simulink model "ZT_VehCtrl_18B"  (R2018b)
settings: Solver=FixedStepAuto  StartTime=0.0  StopTime=inf  FixedStep=0.005  RelTol=1e-3
InitFcn:
  | mbd_mpc_consistency_checks(bdroot(gcs));
undefined symbols (not defined in the file or in its folder): ANG_DEAD, BMS_NormalPwr, BrkPrsByBrkPct_TB_X, BrkPrsByBrkPct_TB_Y, DELAY_DISCHARGE, DELAY_RCUOFF, DRV_BACKWARD, DRV_BRAKE, DRV_FORWARD, DRV_NEUTRAL, DRV_PARK, DRV_UNPARK, DRV_ZEROTURN, EPB_LOCK, EPB_UNLOCK, ExtraLoadPwr, FanOff, fifo_0_vect, fifo_1_vect, HiFanReq, HV_finished, HV_No_Active, HV_POWER_OFF, HV_POWER_ON, HVDown, HVON, KaTLS_v_DrgUp_X_VehSpd, KeFTM_s_Way1OffDlyTime, KeFTM_TK_Way1CoolLv2OffBatTemp, KeFTM_TK_Way1CoolLv2OffMtrTemp, KeFTM_TK_Way1CoolLv2OnBatTemp, KeFTM_TK_Way1CoolLv2OnMtrTemp, KeFTM_TK_Way1CoolLv3OffBatTemp, KeFTM_TK_Way1CoolLv3OffMtrTemp, KeFTM_TK_Way1CoolLv3OnBatTemp, KeFTM_TK_Way1CoolLv3OnMtrTemp, KeFTM_TK_Way1CoolLv4OffBatTemp, KeFTM_TK_Way1CoolLv4OffMtrTemp, KeFTM_TK_Way1CoolLv4OnBatTemp, KeFTM_TK_Way1CoolLv4OnMtrTemp, Kp1, Kp2, LowFanReq, LQFP, MtrPwrFactor_RCU, MtrPwrHighToMidThd, MtrPwrLowToMidThd, MtrPwrMidToHighThd, MtrPwrMidToLowThd, MtrTrqMax, PCT_DEAD, Precharge, PTO_1000, PTO_540, pts1_fifo_0_vect, pts1_fifo_1_vect, pts2_fifo_0_vect, pts2_fifo_1_vect, pts3_fifo_0_vect, pts3_fifo_1_vect ... (+24)
libraries: mbd_mpc574x_ec_toolbox x173, canmsglib x72, simulink x57
(part 5 of 12)

== system ZT_VehCtrl_18B/Initialization & SPI timer1/CS5 LS/Subsystem ==
  Data Store Read : DataStoreRead  DataStoreName=SPIO_CS1_InitFlg
  Merge : Merge  Inputs=3
  Merge1 : Merge  Inputs=3
  SPI_en : Subsystem  TreatAsAtomicUnit=on
  Switch Case : SwitchCase  CaseConditions={1,2,3}  ShowDefaultCase=off
  "clear " : Subsystem  TreatAsAtomicUnit=on
  confi_enbit : Subsystem  TreatAsAtomicUnit=on
  Out1 : Outport
  Out2 : Outport  Port=2
  wires:
  confi_enbit/1(Out1) -> Merge/3
  SPI_en/1(Out1) -> Merge/2
  "clear "/2(Out2) -> Merge1/1
  confi_enbit/2(Out2) -> Merge1/3
  "clear "/1(Out1) -> Merge/1
  Switch Case/1 -> "clear "/Action
  Switch Case/3 -> confi_enbit/Action
  Merge1/1 -> Out2/1
  Switch Case/2 -> SPI_en/Action
  SPI_en/2(Out2) -> Merge1/2
  Data Store Read/1 -> Switch Case/1
  Merge/1 -> Out1/1

== system ZT_VehCtrl_18B/SPI_EEPROM/SPI_write/SPI_enable ==
  Action Port : ActionPort
  Constant1 : Constant  Value=2
  Data Store Write : DataStoreWrite  DataStoreName=Write_Ctrl
  Data Type Conversion : DataTypeConversion  OutDataTypeStr=uint8
  Data Type Conversion3 : DataTypeConversion
  Data Type Conversion8 : DataTypeConversion
  Demux1 : Demux  Outputs=1
  SPI_Master_Transfer_To1 : mbd_mpc574x_ec_toolbox/Communication Blocks/SPI Blocks/SPI_Master_Transfer  Priority=2  InstanceNumber=0  xfermode=Non blocking  timeout=50  spi_upd=on  WhichPCS=0
  Terminator : Terminator
  Vector Concatenate1 : Concatenate  NumInputs=1
  write_enable : Constant  Value=6  OutDataTypeStr=uint8
  wires:
  Data Type Conversion3/1 -> Terminator/1  "r8"
  SPI_Master_Transfer_To1/1 -> Demux1/1
  Demux1/1 -> Data Type Conversion3/1
  Vector Concatenate1/1 -> SPI_Master_Transfer_To1/1
  write_enable/1 -> Data Type Conversion/1
  Data Type Conversion/1 -> Vector Concatenate1/1  "d8"
  Constant1/1 -> Data Type Conversion8/1
  Data Type Conversion8/1 -> Data Store Write/1

== system ZT_VehCtrl_18B/SPI_EEPROM/SPI_write/SPI_write ==
  Action Port : ActionPort
  "Address_High " : Constant  Value=hex2dec('FF')  OutDataTypeStr=uint8
  Address_Low : Constant  Value=hex2dec('FF')
  Constant1 : Constant
  Data Store Read : DataStoreRead  DataStoreName=A_write
  Data Store Write : DataStoreWrite  DataStoreName=Write_Ctrl
  Data Type Conversion{,1..2,5} (4 alike) : DataTypeConversion  OutDataTypeStr=uint8
  Data Type Conversion{3..4,6..8} (5 alike) : DataTypeConversion
  Demux1 : Demux
  SPI_Master_Transfer_To1 : mbd_mpc574x_ec_toolbox/Communication Blocks/SPI Blocks/SPI_Master_Transfer  Priority=2  InstanceNumber=0  xfermode=Non blocking  timeout=50  spi_upd=on  WhichPCS=0
  Terminator{,1..3} (4 alike) : Terminator
  Vector Concatenate1 : Concatenate  NumInputs=4
  write_set : Constant  Value=2  OutDataTypeStr=uint8
  wires:
  Data Type Conversion4/1 -> Terminator1/1  "r5"
  Data Type Conversion3/1 -> Terminator/1  "r4"
  SPI_Master_Transfer_To1/1 -> Demux1/1
  Demux1/1 -> Data Type Conversion3/1
  Vector Concatenate1/1 -> SPI_Master_Transfer_To1/1
  Demux1/2 -> Data Type Conversion4/1
  Address_Low/1 -> Data Type Conversion5/1
  Data Type Conversion/1 -> Vector Concatenate1/1  "d4"
  Data Type Conversion1/1 -> Vector Concatenate1/2  "d5"
  write_set/1 -> Data Type Conversion/1
  "Address_High "/1 -> Data Type Conversion1/1
  Data Store Read/1 -> Data Type Conversion2/1
  Constant1/1 -> Data Type Conversion8/1
  Data Type Conversion5/1 -> Vector Concatenate1/3  "d6"
  Data Type Conversion2/1 -> Vector Concatenate1/4  "d7"
  Data Type Conversion6/1 -> Terminator2/1  "r6"
  Demux1/3 -> Data Type Conversion6/1
  Data Type Conversion7/1 -> Terminator3/1  "r7"
  Demux1/4 -> Data Type Conversion7/1
  Data Type Conversion8/1 -> Data Store Write/1

== system ZT_VehCtrl_18B/SigIn/CAN0 /BMS Cell Battery Temperature ==
  ID : Inport
  Data : Inport  Port=2
  length : Inport  Port=3
  timestamp : Inport  Port=4
  Switch Case : SwitchCase  CaseConditions={hex2dec('357')}  ShowDefaultCase=off
  UNPACK : Subsystem  TreatAsAtomicUnit=on
  Message : Outport
  wires:
  UNPACK/1(Message) -> Message/1
  length/1 -> UNPACK/3(length)
  timestamp/1 -> UNPACK/4(timestamp)
  Data/1 -> UNPACK/2(data)
  ID/1 -> Switch Case/1, UNPACK/1(ID)
  Switch Case/1 -> UNPACK/Action

== system ZT_VehCtrl_18B/SigIn/CAN0 /BMS Cell HeatingTemperature ==
  ID : Inport
  Data : Inport  Port=2
  length : Inport  Port=3
  timestamp : Inport  Port=4
  Switch Case : SwitchCase  CaseConditions={hex2dec('3F3')}  ShowDefaultCase=off
  UNPACK : Subsystem  TreatAsAtomicUnit=on
  Message : Outport
  wires:
  Switch Case/1 -> UNPACK/Action
  ID/1 -> UNPACK/1(ID), Switch Case/1
  Data/1 -> UNPACK/2(data)
  timestamp/1 -> UNPACK/4(timestamp)
  length/1 -> UNPACK/3(length)
  UNPACK/1(Message) -> Message/1

== system ZT_VehCtrl_18B/SigIn/CAN0 /BMS Cell Pole Temperature ==
  ID : Inport
  Data : Inport  Port=2
  length : Inport  Port=3
  timestamp : Inport  Port=4
  Switch Case : SwitchCase  CaseConditions={hex2dec('3F4')}  ShowDefaultCase=off
  UNPACK : Subsystem  TreatAsAtomicUnit=on
  Message : Outport
  wires:
  UNPACK/1(Message) -> Message/1
  length/1 -> UNPACK/3(length)
  timestamp/1 -> UNPACK/4(timestamp)
  Data/1 -> UNPACK/2(data)
  ID/1 -> Switch Case/1, UNPACK/1(ID)
  Switch Case/1 -> UNPACK/Action

== system ZT_VehCtrl_18B/SigIn/CAN0 /BMS Cell Voltage Infor ==
  ID : Inport
  Data : Inport  Port=2
  length : Inport  Port=3
  timestamp : Inport  Port=4
  Switch Case : SwitchCase  CaseConditions={hex2dec('356')}  ShowDefaultCase=off
  UNPACK : Subsystem  TreatAsAtomicUnit=on
  Message : Outport
  wires:
  UNPACK/1(Message) -> Message/1
  length/1 -> UNPACK/3(length)
  timestamp/1 -> UNPACK/4(timestamp)
  Data/1 -> UNPACK/2(data)
  ID/1 -> Switch Case/1, UNPACK/1(ID)
  Switch Case/1 -> UNPACK/Action

== system ZT_VehCtrl_18B/SigIn/CAN0 /BMS CumuCap Infor ==
  ID : Inport
  Data : Inport  Port=2
  length : Inport  Port=3
  timestamp : Inport  Port=4
  Switch Case : SwitchCase  CaseConditions={hex2dec('3F5')}  ShowDefaultCase=off
  UNPACK : Subsystem  TreatAsAtomicUnit=on
  Message : Outport
  wires:
  Switch Case/1 -> UNPACK/Action
  ID/1 -> UNPACK/1(ID), Switch Case/1
  Data/1 -> UNPACK/2(data)
  timestamp/1 -> UNPACK/4(timestamp)
  length/1 -> UNPACK/3(length)
  UNPACK/1(Message) -> Message/1

== system ZT_VehCtrl_18B/SigIn/CAN0 /BMS CumuTimeInfor1 ==
  ID : Inport
  Data : Inport  Port=2
  length : Inport  Port=3
  timestamp : Inport  Port=4
  Switch Case : SwitchCase  CaseConditions={hex2dec('203')}  ShowDefaultCase=off
  UNPACK : Subsystem  TreatAsAtomicUnit=on
  Message : Outport
  wires:
  UNPACK/1(Message) -> Message/1
  length/1 -> UNPACK/3(length)
  timestamp/1 -> UNPACK/4(timestamp)
  Data/1 -> UNPACK/2(data)
  ID/1 -> Switch Case/1, UNPACK/1(ID)
  Switch Case/1 -> UNPACK/Action

== system ZT_VehCtrl_18B/SigIn/CAN0 /BMS CumuTimeInfor2 ==
  ID : Inport
  Data : Inport  Port=2
  length : Inport  Port=3
  timestamp : Inport  Port=4
  Switch Case : SwitchCase  CaseConditions={hex2dec('204')}  ShowDefaultCase=off
  UNPACK : Subsystem  TreatAsAtomicUnit=on
  Message : Outport
  wires:
  Switch Case/1 -> UNPACK/Action
  ID/1 -> UNPACK/1(ID), Switch Case/1
  Data/1 -> UNPACK/2(data)
  timestamp/1 -> UNPACK/4(timestamp)
  length/1 -> UNPACK/3(length)
  UNPACK/1(Message) -> Message/1

== system ZT_VehCtrl_18B/SigIn/CAN0 /BMS HeatInfor ==
  ID : Inport
  Data : Inport  Port=2
  length : Inport  Port=3
  timestamp : Inport  Port=4
  Switch Case : SwitchCase  CaseConditions={hex2dec('208')}  ShowDefaultCase=off
  UNPACK : Subsystem  TreatAsAtomicUnit=on
  Message : Outport
  wires:
  Switch Case/1 -> UNPACK/Action
  ID/1 -> UNPACK/1(ID), Switch Case/1
  Data/1 -> UNPACK/2(data)
  timestamp/1 -> UNPACK/4(timestamp)
  length/1 -> UNPACK/3(length)
  UNPACK/1(Message) -> Message/1

== system ZT_VehCtrl_18B/SigIn/CAN0 /BMS Power Control ==
  ID : Inport
  Data : Inport  Port=2
  length : Inport  Port=3
  timestamp : Inport  Port=4
  Switch Case : SwitchCase  CaseConditions={hex2dec('1F3')}  ShowDefaultCase=off
  UNPACK : Subsystem  TreatAsAtomicUnit=on
  Message : Outport
  wires:
  Switch Case/1 -> UNPACK/Action
  ID/1 -> UNPACK/1(ID), Switch Case/1
  Data/1 -> UNPACK/2(data)
  timestamp/1 -> UNPACK/4(timestamp)
  length/1 -> UNPACK/3(length)
  UNPACK/1(Message) -> Message/1

== system ZT_VehCtrl_18B/SigIn/CAN0 /BMS Power Infor ==
  ID : Inport
  Data : Inport  Port=2
  length : Inport  Port=3
  timestamp : Inport  Port=4
  Switch Case : SwitchCase  CaseConditions={hex2dec('211')}  ShowDefaultCase=off
  UNPACK : Subsystem  TreatAsAtomicUnit=on
  Message : Outport
  wires:
  Switch Case/1 -> UNPACK/Action
  ID/1 -> UNPACK/1(ID), Switch Case/1
  Data/1 -> UNPACK/2(data)
  timestamp/1 -> UNPACK/4(timestamp)
  length/1 -> UNPACK/3(length)
  UNPACK/1(Message) -> Message/1

== system ZT_VehCtrl_18B/SigIn/CAN0 /BMS StartDia_Infor1 ==
  ID : Inport
  Data : Inport  Port=2
  length : Inport  Port=3
  timestamp : Inport  Port=4
  Switch Case : SwitchCase  CaseConditions={hex2dec('206')}  ShowDefaultCase=off
  UNPACK : Subsystem  TreatAsAtomicUnit=on
  Message : Outport
  wires:
  Switch Case/1 -> UNPACK/Action
  ID/1 -> UNPACK/1(ID), Switch Case/1
  Data/1 -> UNPACK/2(data)
  timestamp/1 -> UNPACK/4(timestamp)
  length/1 -> UNPACK/3(length)
  UNPACK/1(Message) -> Message/1

== system ZT_VehCtrl_18B/SigIn/CAN0 /BMS StartDia_Infor2 ==
  ID : Inport
  Data : Inport  Port=2
  length : Inport  Port=3
  timestamp : Inport  Port=4
  Switch Case : SwitchCase  CaseConditions={hex2dec('207')}  ShowDefaultCase=off
  UNPACK : Subsystem  TreatAsAtomicUnit=on
  Message : Outport
  wires:
  UNPACK/1(Message) -> Message/1
  length/1 -> UNPACK/3(length)
  timestamp/1 -> UNPACK/4(timestamp)
  Data/1 -> UNPACK/2(data)
  ID/1 -> Switch Case/1, UNPACK/1(ID)
  Switch Case/1 -> UNPACK/Action

== system ZT_VehCtrl_18B/SigIn/CAN0 /BMS Statistic_Cell ExtremumIndex Infor ==
  ID : Inport
  Data : Inport  Port=2
  length : Inport  Port=3
  timestamp : Inport  Port=4
  Switch Case : SwitchCase  CaseConditions={hex2dec('358')}  ShowDefaultCase=off
  UNPACK : Subsystem  TreatAsAtomicUnit=on
  Message : Outport
  wires:
  UNPACK/1(Message) -> Message/1
  length/1 -> UNPACK/3(length)
  timestamp/1 -> UNPACK/4(timestamp)
  Data/1 -> UNPACK/2(data)
  ID/1 -> Switch Case/1, UNPACK/1(ID)
  Switch Case/1 -> UNPACK/Action

== system ZT_VehCtrl_18B/SigIn/CAN0 /BMS Statistic_Cell Voltage Infor ==
  ID : Inport
  Data : Inport  Port=2
  length : Inport  Port=3
  timestamp : Inport  Port=4
  Switch Case : SwitchCase  CaseConditions={hex2dec('352')}  ShowDefaultCase=off
  UNPACK : Subsystem  TreatAsAtomicUnit=on
  Message : Outport
  wires:
  UNPACK/1(Message) -> Message/1
  length/1 -> UNPACK/3(length)
  timestamp/1 -> UNPACK/4(timestamp)
  Data/1 -> UNPACK/2(data)
  ID/1 -> Switch Case/1, UNPACK/1(ID)
  Switch Case/1 -> UNPACK/Action

== system ZT_VehCtrl_18B/SigIn/CAN0 /BMS Statistic_HeatingTemperature ==
  ID : Inport
  Data : Inport  Port=2
  length : Inport  Port=3
  timestamp : Inport  Port=4
  Switch Case : SwitchCase  CaseConditions={hex2dec('354')}  ShowDefaultCase=off
  UNPACK : Subsystem  TreatAsAtomicUnit=on
  Message : Outport
  wires:
  UNPACK/1(Message) -> Message/1
  length/1 -> UNPACK/3(length)
  timestamp/1 -> UNPACK/4(timestamp)
  Data/1 -> UNPACK/2(data)
  ID/1 -> Switch Case/1, UNPACK/1(ID)
  Switch Case/1 -> UNPACK/Action

== system ZT_VehCtrl_18B/SigIn/CAN0 /BMS Statistic_PoleTemperature ==
  ID : Inport
  Data : Inport  Port=2
  length : Inport  Port=3
  timestamp : Inport  Port=4
  Switch Case : SwitchCase  CaseConditions={hex2dec('355')}  ShowDefaultCase=off
  UNPACK : Subsystem  TreatAsAtomicUnit=on
  Message : Outport
  wires:
  UNPACK/1(Message) -> Message/1
  length/1 -> UNPACK/3(length)
  timestamp/1 -> UNPACK/4(timestamp)
  Data/1 -> UNPACK/2(data)
  ID/1 -> Switch Case/1, UNPACK/1(ID)
  Switch Case/1 -> UNPACK/Action

== system ZT_VehCtrl_18B/SigIn/CAN0 /BMS Statistic_Temperature of Battery ==
  ID : Inport
  Data : Inport  Port=2
  length : Inport  Port=3
  timestamp : Inport  Port=4
  Switch Case : SwitchCase  CaseConditions={hex2dec('353')}  ShowDefaultCase=off
  UNPACK : Subsystem  TreatAsAtomicUnit=on
  Message : Outport
  wires:
  UNPACK/1(Message) -> Message/1
  length/1 -> UNPACK/3(length)
  timestamp/1 -> UNPACK/4(timestamp)
  Data/1 -> UNPACK/2(data)
  ID/1 -> Switch Case/1, UNPACK/1(ID)
  Switch Case/1 -> UNPACK/Action

== system ZT_VehCtrl_18B/SigIn/CAN0 /BMS _SystemTime  ==
  ID : Inport
  Data : Inport  Port=2
  length : Inport  Port=3
  timestamp : Inport  Port=4
  Switch Case : SwitchCase  CaseConditions={hex2dec('202')}  ShowDefaultCase=off
  UNPACK : Subsystem  TreatAsAtomicUnit=on
  Message : Outport
  wires:
  Switch Case/1 -> UNPACK/Action
  ID/1 -> UNPACK/1(ID), Switch Case/1
  Data/1 -> UNPACK/2(data)
  timestamp/1 -> UNPACK/4(timestamp)
  length/1 -> UNPACK/3(length)
  UNPACK/1(Message) -> Message/1

== system ZT_VehCtrl_18B/SigIn/CAN0 /BMS other Information1 ==
  ID : Inport
  Data : Inport  Port=2
  length : Inport  Port=3
  timestamp : Inport  Port=4
  Switch Case : SwitchCase  CaseConditions={hex2dec('3F6')}  ShowDefaultCase=off
  UNPACK : Subsystem  TreatAsAtomicUnit=on
  Message : Outport
  wires:
  UNPACK/1(Message) -> Message/1
  length/1 -> UNPACK/3(length)
  timestamp/1 -> UNPACK/4(timestamp)
  Data/1 -> UNPACK/2(data)
  ID/1 -> Switch Case/1, UNPACK/1(ID)
  Switch Case/1 -> UNPACK/Action

== system ZT_VehCtrl_18B/SigIn/CAN0 /BMS other Information2  ==
  ID : Inport
  Data : Inport  Port=2
  length : Inport  Port=3
  timestamp : Inport  Port=4
  Switch Case : SwitchCase  CaseConditions={hex2dec('3FF')}  ShowDefaultCase=off
  UNPACK : Subsystem  TreatAsAtomicUnit=on
  Message : Outport
  wires:
  Switch Case/1 -> UNPACK/Action
  ID/1 -> UNPACK/1(ID), Switch Case/1
  Data/1 -> UNPACK/2(data)
  timestamp/1 -> UNPACK/4(timestamp)
  length/1 -> UNPACK/3(length)
  UNPACK/1(Message) -> Message/1

== system ZT_VehCtrl_18B/SigIn/CAN0 /BMS other Information3 ==
  ID : Inport
  Data : Inport  Port=2
  length : Inport  Port=3
  timestamp : Inport  Port=4
  Switch Case : SwitchCase  CaseConditions={hex2dec('205')}  ShowDefaultCase=off
  UNPACK : Subsystem  TreatAsAtomicUnit=on
  Message : Outport
  wires:
  UNPACK/1(Message) -> Message/1
  length/1 -> UNPACK/3(length)
  timestamp/1 -> UNPACK/4(timestamp)
  Data/1 -> UNPACK/2(data)
  ID/1 -> Switch Case/1, UNPACK/1(ID)
  Switch Case/1 -> UNPACK/Action

== system ZT_VehCtrl_18B/SigIn/CAN0 /BMSWarning_Status ==
  ID : Inport
  Data : Inport  Port=2
  length : Inport  Port=3
  timestamp : Inport  Port=4
  Switch Case : SwitchCase  CaseConditions={hex2dec('1F5')}  ShowDefaultCase=off
  UNPACK : Subsystem  TreatAsAtomicUnit=on
  Message : Outport
  wires:
  UNPACK/1(Message) -> Message/1
  length/1 -> UNPACK/3(length)
  timestamp/1 -> UNPACK/4(timestamp)
  Data/1 -> UNPACK/2(data)
  ID/1 -> Switch Case/1, UNPACK/1(ID)
  Switch Case/1 -> UNPACK/Action

== system ZT_VehCtrl_18B/SigIn/CAN0 /BMS_Information1 ==
  ID : Inport
  Data : Inport  Port=2
  length : Inport  Port=3
  timestamp : Inport  Port=4
  Switch Case : SwitchCase  CaseConditions={hex2dec('1E1')}  ShowDefaultCase=off
  UNPACK : Subsystem  TreatAsAtomicUnit=on
  Message : Outport
  wires:
  UNPACK/1(Message) -> Message/1
  length/1 -> UNPACK/3(length)
  timestamp/1 -> UNPACK/4(timestamp)
  Data/1 -> UNPACK/2(data)
  ID/1 -> Switch Case/1, UNPACK/1(ID)
  Switch Case/1 -> UNPACK/Action

== system ZT_VehCtrl_18B/SigIn/CAN0 /BMS_Information2 ==
  ID : Inport
  Data : Inport  Port=2
  length : Inport  Port=3
  timestamp : Inport  Port=4
  Switch Case : SwitchCase  CaseConditions={hex2dec('1E4')}  ShowDefaultCase=off
  UNPACK : Subsystem  TreatAsAtomicUnit=on
  Message : Outport
  wires:
  Switch Case/1 -> UNPACK/Action
  ID/1 -> UNPACK/1(ID), Switch Case/1
  Data/1 -> UNPACK/2(data)
  timestamp/1 -> UNPACK/4(timestamp)
  length/1 -> UNPACK/3(length)
  UNPACK/1(Message) -> Message/1

== system ZT_VehCtrl_18B/SigIn/CAN0 /BMS_Relay Status ==
  ID : Inport
  Data : Inport  Port=2
  length : Inport  Port=3
  timestamp : Inport  Port=4
  Switch Case : SwitchCase  CaseConditions={hex2dec('351')}  ShowDefaultCase=off
  UNPACK : Subsystem  TreatAsAtomicUnit=on
  Message : Outport
  wires:
  UNPACK/1(Message) -> Message/1
  length/1 -> UNPACK/3(length)
  timestamp/1 -> UNPACK/4(timestamp)
  Data/1 -> UNPACK/2(data)
  ID/1 -> Switch Case/1, UNPACK/1(ID)
  Switch Case/1 -> UNPACK/Action

== system ZT_VehCtrl_18B/SigIn/CAN0 /BMS_Relay Status2 ==
  ID : Inport
  Data : Inport  Port=2
  length : Inport  Port=3
  timestamp : Inport  Port=4
  Switch Case : SwitchCase  CaseConditions={hex2dec('360')}  ShowDefaultCase=off
  UNPACK : Subsystem  TreatAsAtomicUnit=on
  Message : Outport
  wires:
  UNPACK/1(Message) -> Message/1
  length/1 -> UNPACK/3(length)
  timestamp/1 -> UNPACK/4(timestamp)
  Data/1 -> UNPACK/2(data)
  ID/1 -> Switch Case/1, UNPACK/1(ID)
  Switch Case/1 -> UNPACK/Action

== system ZT_VehCtrl_18B/SigIn/CAN0 /BMS_Relay Status3 ==
  ID : Inport
  Data : Inport  Port=2
  length : Inport  Port=3
  timestamp : Inport  Port=4
  Switch Case : SwitchCase  CaseConditions={hex2dec('361')}  ShowDefaultCase=off
  UNPACK : Subsystem  TreatAsAtomicUnit=on
  Message : Outport
  wires:
  Switch Case/1 -> UNPACK/Action
  ID/1 -> UNPACK/1(ID), Switch Case/1
  Data/1 -> UNPACK/2(data)
  timestamp/1 -> UNPACK/4(timestamp)
  length/1 -> UNPACK/3(length)
  UNPACK/1(Message) -> Message/1

== system ZT_VehCtrl_18B/SigIn/CAN0 /BRS2VCU1 ==
  ID : Inport
  Data : Inport  Port=2
  length : Inport  Port=3
  timestamp : Inport  Port=4
  Switch Case : SwitchCase  CaseConditions={hex2dec('18FE25E4')}  ShowDefaultCase=off
  UNPACK : Subsystem  TreatAsAtomicUnit=on
  Message : Outport
  wires:
  Switch Case/1 -> UNPACK/Action
  ID/1 -> UNPACK/1(ID), Switch Case/1
  Data/1 -> UNPACK/2(data)
  timestamp/1 -> UNPACK/4(timestamp)
  length/1 -> UNPACK/3(length)
  UNPACK/1(Message) -> Message/1

== system ZT_VehCtrl_18B/SigIn/CAN0 /BRS2VCU2 ==
  ID : Inport
  Data : Inport  Port=2
  length : Inport  Port=3
  timestamp : Inport  Port=4
  Switch Case : SwitchCase  CaseConditions={hex2dec('18FE26E4')}  ShowDefaultCase=off
  UNPACK : Subsystem  TreatAsAtomicUnit=on
  Message : Outport
  wires:
  UNPACK/1(Message) -> Message/1
  length/1 -> UNPACK/3(length)
  timestamp/1 -> UNPACK/4(timestamp)
  Data/1 -> UNPACK/2(data)
  ID/1 -> Switch Case/1, UNPACK/1(ID)
  Switch Case/1 -> UNPACK/Action

== system ZT_VehCtrl_18B/SigIn/CAN0 /BRS2VCU3 ==
  ID : Inport
  Data : Inport  Port=2
  length : Inport  Port=3
  timestamp : Inport  Port=4
  Switch Case : SwitchCase  CaseConditions={hex2dec('18FE27E4')}  ShowDefaultCase=off
  UNPACK : Subsystem  TreatAsAtomicUnit=on
  Message : Outport
  wires:
  Switch Case/1 -> UNPACK/Action
  ID/1 -> UNPACK/1(ID), Switch Case/1
  Data/1 -> UNPACK/2(data)
  timestamp/1 -> UNPACK/4(timestamp)
  length/1 -> UNPACK/3(length)
  UNPACK/1(Message) -> Message/1

== system ZT_VehCtrl_18B/SigIn/CAN0 /OBC_Charger Status ==
  ID : Inport
  Data : Inport  Port=2
  length : Inport  Port=3
  timestamp : Inport  Port=4
  Switch Case : SwitchCase  CaseConditions={hex2dec('220')}  ShowDefaultCase=off
  UNPACK : Subsystem  TreatAsAtomicUnit=on
  Message : Outport
  wires:
  Switch Case/1 -> UNPACK/Action
  ID/1 -> UNPACK/1(ID), Switch Case/1
  Data/1 -> UNPACK/2(data)
  timestamp/1 -> UNPACK/4(timestamp)
  length/1 -> UNPACK/3(length)
  UNPACK/1(Message) -> Message/1

== system ZT_VehCtrl_18B/SigIn/CAN0 /TMS2VCU ==
  ID : Inport
  Data : Inport  Port=2
  length : Inport  Port=3
  timestamp : Inport  Port=4
  Switch Case : SwitchCase  CaseConditions={hex2dec('18FFF346')}  ShowDefaultCase=off
  UNPACK : Subsystem  TreatAsAtomicUnit=on
  Message : Outport
  wires:
  UNPACK/1(Message) -> Message/1
  length/1 -> UNPACK/3(length)
  timestamp/1 -> UNPACK/4(timestamp)
  Data/1 -> UNPACK/2(data)
  ID/1 -> Switch Case/1, UNPACK/1(ID)
  Switch Case/1 -> UNPACK/Action

== system ZT_VehCtrl_18B/SigIn/CAN1/ACU1 ==
  ID : Inport
  Data : Inport  Port=2
  length : Inport  Port=3
  timestamp : Inport  Port=4
  Switch Case : SwitchCase  CaseConditions={hex2dec('0C08A79A')}  ShowDefaultCase=off
  UNPACK : Subsystem  TreatAsAtomicUnit=on
  Message : Outport
  wires:
  Switch Case/1 -> UNPACK/Action
  ID/1 -> UNPACK/1(ID), Switch Case/1
  Data/1 -> UNPACK/2(data)
  timestamp/1 -> UNPACK/4(timestamp)
  length/1 -> UNPACK/3(length)
  UNPACK/1(Message) -> Message/1

== system ZT_VehCtrl_18B/SigIn/CAN1/ACU2 ==
  ID : Inport
  Data : Inport  Port=2
  length : Inport  Port=3
  timestamp : Inport  Port=4
  Switch Case : SwitchCase  CaseConditions={hex2dec('0C09A79B')}  ShowDefaultCase=off
  UNPACK : Subsystem  TreatAsAtomicUnit=on
  Message : Outport
  wires:
  UNPACK/1(Message) -> Message/1
  length/1 -> UNPACK/3(length)
  timestamp/1 -> UNPACK/4(timestamp)
  Data/1 -> UNPACK/2(data)
  ID/1 -> Switch Case/1, UNPACK/1(ID)
  Switch Case/1 -> UNPACK/Action

== system ZT_VehCtrl_18B/SigIn/CAN1/ACU3 ==
  ID : Inport
  Data : Inport  Port=2
  length : Inport  Port=3
  timestamp : Inport  Port=4
  Switch Case : SwitchCase  CaseConditions={hex2dec('0C0AA79D')}  ShowDefaultCase=off
  UNPACK : Subsystem  TreatAsAtomicUnit=on
  Message : Outport
  wires:
  Switch Case/1 -> UNPACK/Action
  ID/1 -> UNPACK/1(ID), Switch Case/1
  Data/1 -> UNPACK/2(data)
  timestamp/1 -> UNPACK/4(timestamp)
  length/1 -> UNPACK/3(length)
  UNPACK/1(Message) -> Message/1

== system ZT_VehCtrl_18B/SigIn/CAN1/HVC1_LV ==
  ID : Inport
  Data : Inport  Port=2
  length : Inport  Port=3
  timestamp : Inport  Port=4
  Switch Case : SwitchCase  CaseConditions={hex2dec('180105A1')}  ShowDefaultCase=off
  UNPACK : Subsystem  TreatAsAtomicUnit=on
  Message : Outport
  wires:
  Switch Case/1 -> UNPACK/Action
  ID/1 -> UNPACK/1(ID), Switch Case/1
  Data/1 -> UNPACK/2(data)
  timestamp/1 -> UNPACK/4(timestamp)
  length/1 -> UNPACK/3(length)
  UNPACK/1(Message) -> Message/1

== system ZT_VehCtrl_18B/SigIn/CAN1/HVC3_Temp ==
  ID : Inport
  Data : Inport  Port=2
  length : Inport  Port=3
  timestamp : Inport  Port=4
  Switch Case : SwitchCase  CaseConditions={hex2dec('180305A1')}  ShowDefaultCase=off
  UNPACK : Subsystem  TreatAsAtomicUnit=on
  Message : Outport
  wires:
  UNPACK/1(Message) -> Message/1
  length/1 -> UNPACK/3(length)
  timestamp/1 -> UNPACK/4(timestamp)
  Data/1 -> UNPACK/2(data)
  ID/1 -> Switch Case/1, UNPACK/1(ID)
  Switch Case/1 -> UNPACK/Action

== system ZT_VehCtrl_18B/SigIn/CAN1/HVC4_RlySt ==
  ID : Inport
  Data : Inport  Port=2
  length : Inport  Port=3
  timestamp : Inport  Port=4
  Switch Case : SwitchCase  CaseConditions={hex2dec('180405A1')}  ShowDefaultCase=off
  UNPACK : Subsystem  TreatAsAtomicUnit=on
  Message : Outport
  wires:
  Switch Case/1 -> UNPACK/Action
  ID/1 -> UNPACK/1(ID), Switch Case/1
  Data/1 -> UNPACK/2(data)
  timestamp/1 -> UNPACK/4(timestamp)
  length/1 -> UNPACK/3(length)
  UNPACK/1(Message) -> Message/1

== system ZT_VehCtrl_18B/SigIn/CAN1/HVC7_HV1 ==
  ID : Inport
  Data : Inport  Port=2
  length : Inport  Port=3
  timestamp : Inport  Port=4
  Switch Case : SwitchCase  CaseConditions={hex2dec('180705A1')}  ShowDefaultCase=off
  UNPACK : Subsystem  TreatAsAtomicUnit=on
  Message : Outport
  wires:
  UNPACK/1(Message) -> Message/1
  length/1 -> UNPACK/3(length)
  timestamp/1 -> UNPACK/4(timestamp)
  Data/1 -> UNPACK/2(data)
  ID/1 -> Switch Case/1, UNPACK/1(ID)
  Switch Case/1 -> UNPACK/Action

== system ZT_VehCtrl_18B/SigIn/CAN1/ISG MCU STATUS 1 ==
  ID : Inport
  Data : Inport  Port=2
  length : Inport  Port=3
  timestamp : Inport  Port=4
  Switch Case : SwitchCase  CaseConditions={hex2dec('CFF0006')}  ShowDefaultCase=off
  UNPACK : Subsystem  TreatAsAtomicUnit=on
  Message : Outport
  wires:
  Switch Case/1 -> UNPACK/Action
  ID/1 -> UNPACK/1(ID), Switch Case/1
  Data/1 -> UNPACK/2(data)
  timestamp/1 -> UNPACK/4(timestamp)
  length/1 -> UNPACK/3(length)
  UNPACK/1(Message) -> Message/1

== system ZT_VehCtrl_18B/SigIn/CAN1/ISG MCU STATUS 2 ==
  ID : Inport
  Data : Inport  Port=2
  length : Inport  Port=3
  timestamp : Inport  Port=4
  Switch Case : SwitchCase  CaseConditions={hex2dec('CFF0106')}  ShowDefaultCase=off
  UNPACK : Subsystem  TreatAsAtomicUnit=on
  Message : Outport
  wires:
  UNPACK/1(Message) -> Message/1
  length/1 -> UNPACK/3(length)
  timestamp/1 -> UNPACK/4(timestamp)
  Data/1 -> UNPACK/2(data)
  ID/1 -> Switch Case/1, UNPACK/1(ID)
  Switch Case/1 -> UNPACK/Action

== system ZT_VehCtrl_18B/SigIn/CAN1/ISG MCU STATUS 3 ==
  ID : Inport
  Data : Inport  Port=2
  length : Inport  Port=3
  timestamp : Inport  Port=4
  Switch Case : SwitchCase  CaseConditions={hex2dec('CFF0206')}  ShowDefaultCase=off
  UNPACK : Subsystem  TreatAsAtomicUnit=on
  Message : Outport
  wires:
  Switch Case/1 -> UNPACK/Action
  ID/1 -> UNPACK/1(ID), Switch Case/1
  Data/1 -> UNPACK/2(data)
  timestamp/1 -> UNPACK/4(timestamp)
  length/1 -> UNPACK/3(length)
  UNPACK/1(Message) -> Message/1

== system ZT_VehCtrl_18B/SigIn/CAN1/MCU1Msg1 ==
  ID : Inport
  Data : Inport  Port=2
  length : Inport  Port=3
  timestamp : Inport  Port=4
  Switch Case : SwitchCase  CaseConditions={hex2dec('1836D0EF')}  ShowDefaultCase=off
  UNPACK : Subsystem  TreatAsAtomicUnit=on
  Message : Outport
  wires:
  UNPACK/1(Message) -> Message/1
  length/1 -> UNPACK/3(length)
  timestamp/1 -> UNPACK/4(timestamp)
  Data/1 -> UNPACK/2(data)
  ID/1 -> Switch Case/1, UNPACK/1(ID)
  Switch Case/1 -> UNPACK/Action

== system ZT_VehCtrl_18B/SigIn/CAN1/MCU1Msg2 ==
  ID : Inport
  Data : Inport  Port=2
  length : Inport  Port=3
  timestamp : Inport  Port=4
  Switch Case : SwitchCase  CaseConditions={hex2dec('1837D0EF')}  ShowDefaultCase=off
  UNPACK : Subsystem  TreatAsAtomicUnit=on
  Message : Outport
  wires:
  Switch Case/1 -> UNPACK/Action
  ID/1 -> UNPACK/1(ID), Switch Case/1
  Data/1 -> UNPACK/2(data)
  timestamp/1 -> UNPACK/4(timestamp)
  length/1 -> UNPACK/3(length)
  UNPACK/1(Message) -> Message/1

== system ZT_VehCtrl_18B/SigIn/CAN1/MCU1Msg3 ==
  ID : Inport
  Data : Inport  Port=2
  length : Inport  Port=3
  timestamp : Inport  Port=4
  Switch Case : SwitchCase  CaseConditions={hex2dec('1838D0EF')}  ShowDefaultCase=off
  UNPACK : Subsystem  TreatAsAtomicUnit=on
  Message : Outport
  wires:
  UNPACK/1(Message) -> Message/1
  length/1 -> UNPACK/3(length)
  timestamp/1 -> UNPACK/4(timestamp)
  Data/1 -> UNPACK/2(data)
  ID/1 -> Switch Case/1, UNPACK/1(ID)
  Switch Case/1 -> UNPACK/Action

== system ZT_VehCtrl_18B/SigIn/CAN1/MCU2Msg1 ==
  ID : Inport
  Data : Inport  Port=2
  length : Inport  Port=3
  timestamp : Inport  Port=4
  Switch Case : SwitchCase  CaseConditions={hex2dec('1836D0F1')}  ShowDefaultCase=off
  UNPACK : Subsystem  TreatAsAtomicUnit=on
  Message : Outport
  wires:
  Switch Case/1 -> UNPACK/Action
  ID/1 -> UNPACK/1(ID), Switch Case/1
  Data/1 -> UNPACK/2(data)
  timestamp/1 -> UNPACK/4(timestamp)
  length/1 -> UNPACK/3(length)
  UNPACK/1(Message) -> Message/1

== system ZT_VehCtrl_18B/SigIn/CAN1/MCU2Msg2 ==
  ID : Inport
  Data : Inport  Port=2
  length : Inport  Port=3
  timestamp : Inport  Port=4
  Switch Case : SwitchCase  CaseConditions={hex2dec('1837D0F1')}  ShowDefaultCase=off
  UNPACK : Subsystem  TreatAsAtomicUnit=on
  Message : Outport
  wires:
  UNPACK/1(Message) -> Message/1
  length/1 -> UNPACK/3(length)
  timestamp/1 -> UNPACK/4(timestamp)
  Data/1 -> UNPACK/2(data)
  ID/1 -> Switch Case/1, UNPACK/1(ID)
  Switch Case/1 -> UNPACK/Action

== system ZT_VehCtrl_18B/SigIn/CAN1/MCU2Msg3 ==
  ID : Inport
  Data : Inport  Port=2
  length : Inport  Port=3
  timestamp : Inport  Port=4
  Switch Case : SwitchCase  CaseConditions={hex2dec('1838D0F1')}  ShowDefaultCase=off
  UNPACK : Subsystem  TreatAsAtomicUnit=on
  Message : Outport
  wires:
  Switch Case/1 -> UNPACK/Action
  ID/1 -> UNPACK/1(ID), Switch Case/1
  Data/1 -> UNPACK/2(data)
  timestamp/1 -> UNPACK/4(timestamp)
  length/1 -> UNPACK/3(length)
  UNPACK/1(Message) -> Message/1

== system ZT_VehCtrl_18B/SigIn/CAN1/PDU_RelaySts ==
  ID : Inport
  Data : Inport  Port=2
  length : Inport  Port=3
  timestamp : Inport  Port=4
  Switch Case : SwitchCase  CaseConditions={hex2dec('18FF2BC8')}  ShowDefaultCase=off
  UNPACK : Subsystem  TreatAsAtomicUnit=on
  Message : Outport
  wires:
  UNPACK/1(Message) -> Message/1
  length/1 -> UNPACK/3(length)
  timestamp/1 -> UNPACK/4(timestamp)
  Data/1 -> UNPACK/2(data)
  ID/1 -> Switch Case/1, UNPACK/1(ID)
  Switch Case/1 -> UNPACK/Action

== system ZT_VehCtrl_18B/SigIn/CAN1/TM MCU STATUS 1 ==
  ID : Inport
  Data : Inport  Port=2
  length : Inport  Port=3
  timestamp : Inport  Port=4
  Switch Case : SwitchCase  CaseConditions={hex2dec('CFF0005')}  ShowDefaultCase=off
  UNPACK : Subsystem  TreatAsAtomicUnit=on
  Message : Outport
  wires:
  UNPACK/1(Message) -> Message/1
  length/1 -> UNPACK/3(length)
  timestamp/1 -> UNPACK/4(timestamp)
  Data/1 -> UNPACK/2(data)
  ID/1 -> Switch Case/1, UNPACK/1(ID)
  Switch Case/1 -> UNPACK/Action

== system ZT_VehCtrl_18B/SigIn/CAN1/TM MCU STATUS 2 ==
  ID : Inport
  Data : Inport  Port=2
  length : Inport  Port=3
  timestamp : Inport  Port=4
  Switch Case : SwitchCase  CaseConditions={hex2dec('CFF0105')}  ShowDefaultCase=off
  UNPACK : Subsystem  TreatAsAtomicUnit=on
  Message : Outport
  wires:
  Switch Case/1 -> UNPACK/Action
  ID/1 -> UNPACK/1(ID), Switch Case/1
  Data/1 -> UNPACK/2(data)
  timestamp/1 -> UNPACK/4(timestamp)
  length/1 -> UNPACK/3(length)
  UNPACK/1(Message) -> Message/1

== system ZT_VehCtrl_18B/SigIn/CAN1/TM MCU STATUS 3 ==
  ID : Inport
  Data : Inport  Port=2
  length : Inport  Port=3
  timestamp : Inport  Port=4
  Switch Case : SwitchCase  CaseConditions={hex2dec('CFF0205')}  ShowDefaultCase=off
  UNPACK : Subsystem  TreatAsAtomicUnit=on
  Message : Outport
  wires:
  UNPACK/1(Message) -> Message/1
  length/1 -> UNPACK/3(length)
  timestamp/1 -> UNPACK/4(timestamp)
  Data/1 -> UNPACK/2(data)
  ID/1 -> Switch Case/1, UNPACK/1(ID)
  Switch Case/1 -> UNPACK/Action

== system ZT_VehCtrl_18B/SigIn/CAN1/TWV  ==
  ID : Inport
  Data : Inport  Port=2
  length : Inport  Port=3
  timestamp : Inport  Port=4
  Switch Case : SwitchCase  CaseConditions={hex2dec('18FF243B')}  ShowDefaultCase=off
  UNPACK : Subsystem  TreatAsAtomicUnit=on
  Message : Outport
  wires:
  Switch Case/1 -> UNPACK/Action
  ID/1 -> UNPACK/1(ID), Switch Case/1
  Data/1 -> UNPACK/2(data)
  timestamp/1 -> UNPACK/4(timestamp)
  length/1 -> UNPACK/3(length)
  UNPACK/1(Message) -> Message/1

== system ZT_VehCtrl_18B/SigIn/DI/DI_31_32_33_34 ==
  note: DI PWM PULLUP
  note: DI PWM PULLDOWN
  DI31 : mbd_mpc574x_ec_toolbox/GPIO Blocks/Digital_Input  gpio_pin=PTF0: [SIUL2_GPIO80 | General Purpose IO PF[0]]  pull_resistor=None
  DI32 : mbd_mpc574x_ec_toolbox/GPIO Blocks/Digital_Input  gpio_pin=PTD1: [SIUL2_GPIO49 | General Purpose IO PD[1]]  pull_resistor=None
  DI33 : mbd_mpc574x_ec_toolbox/GPIO Blocks/Digital_Input  gpio_pin=PTD2: [SIUL2_GPIO50 | General Purpose IO PD[2]]  pull_resistor=None
  DI34 : mbd_mpc574x_ec_toolbox/GPIO Blocks/Digital_Input  gpio_pin=PTC13: [SIUL2_GPIO45 | General Purpose IO PC[13]]  pull_resistor=None
  Data Store Write14 : DataStoreWrite  DataStoreName=DI31
  Data Store Write15 : DataStoreWrite  DataStoreName=DI32
  Data Store Write16 : DataStoreWrite  DataStoreName=DI33
  Data Store Write17 : DataStoreWrite  DataStoreName=DI34
  wires:
  DI34/1 -> Data Store Write17/1
  DI33/1 -> Data Store Write16/1
  DI32/1 -> Data Store Write15/1
  DI31/1 -> Data Store Write14/1

== system ZT_VehCtrl_18B/SigIn/PWM/PWM_PTS1 ==
  Add : Sum  Inputs=+-  AccumDataTypeStr=single
  Add1 : Sum  Inputs=+-  AccumDataTypeStr=single
  Data Store Memory : DataStoreMemory  DataStoreName=pts1_pwm_cnt  ReadBeforeWriteMsg=warning  WriteAfterWriteMsg=warning  WriteAfterReadMsg=warning  ShowAdditionalParam=off  OutDataTypeStr=uint8
  Data Store Memory2 : DataStoreMemory  DataStoreName=pts1_fifo_1_vect  ReadBeforeWriteMsg=warning  WriteAfterWriteMsg=warning  WriteAfterReadMsg=warning  InitialValue=[0 0 0 0 0 0 0 0]  ShowAdditionalParam=off  OutDataTypeStr=uint16
  Data Store Memory4 : DataStoreMemory  DataStoreName=pts1_fifo_0_vect  ReadBeforeWriteMsg=warning  WriteAfterWriteMsg=warning  WriteAfterReadMsg=warning  InitialValue=[0 0 0 0 0 0 0 0]  ShowAdditionalParam=off  OutDataTypeStr=uint16
  Data Store Read : DataStoreRead  DataStoreName=pts1_fifo_0_vect  DataStoreElements=pts1_fifo_0_vect(2)#pts1_fifo_0_vect(1)
  Data Store Read1 : DataStoreRead  DataStoreName=pts1_fifo_1_vect  DataStoreElements=pts1_fifo_1_vect(1)
  Data Store Read2 : DataStoreRead  DataStoreName=pts1_fifo_0_vect  DataStoreElements=pts1_fifo_0_vect(1)
  Data Store Write3 : DataStoreWrite  DataStoreName=pts1_fifo_0_vect
  Data Store Write5 : DataStoreWrite  DataStoreName=pts1_fifo_1_vect
  Divide : Product  Inputs=*/  OutDataTypeStr=single
  Divide1 : Product  Inputs=*//
  Freq_MC : Constant  Value=80000000  OutDataTypeStr=single
  Prescaler : Constant  Value=32  OutDataTypeStr=single
  Subsystem : Subsystem
  Subsystem_capture : Subsystem
  Terminator1 : Terminator
  Terminator2 : Terminator
  eTimer_ISR : mbd_mpc574x_ec_toolbox/Motor Control Blocks/eTIMER Blocks/eTimer_ISR_Handler  etimerModule=1  etimerInterrupt=Channel Interrupt  etimerChannel=2  etimerIsrPriority=14
      settings: SourceProductName=NXP Model-Based Design Toolbox for MPC57xx MCUs
  DC : Outport
  freq : Outport  Port=2
  wires:
  eTimer_ISR/2 -> Subsystem_capture/1(In1)
  Subsystem_capture/1(Out1) -> Terminator1/1
  Subsystem_capture/3(Out3) -> Terminator2/1
  Subsystem_capture/4(Out4) -> Data Store Write5/1
  Subsystem_capture/2(Out2) -> Data Store Write3/1
  eTimer_ISR/1 -> Subsystem_capture/Trigger
  Prescaler/1 -> Divide1/2
  Add/1 -> Divide/2, Divide1/3
  Data Store Read1/1 -> Add1/1
  Data Store Read/2 -> Add/2
  Freq_MC/1 -> Divide1/1
  Add1/1 -> Divide/1
  Data Store Read2/1 -> Add1/2
  Divide1/1 -> freq/1
  Data Store Read/1 -> Add/1
  Divide/1 -> Subsystem/1(In1)
  Subsystem/1(Out1) -> DC/1

== system ZT_VehCtrl_18B/SigIn/PWM/PWM_PTS2 ==
  Add : Sum  Inputs=+-  AccumDataTypeStr=single
  Add1 : Sum  Inputs=+-  AccumDataTypeStr=single
  Data Store Memory : DataStoreMemory  DataStoreName=pts2_pwm_cnt  ReadBeforeWriteMsg=warning  WriteAfterWriteMsg=warning  WriteAfterReadMsg=warning  ShowAdditionalParam=off  OutDataTypeStr=uint8
  Data Store Memory2 : DataStoreMemory  DataStoreName=pts2_fifo_1_vect  ReadBeforeWriteMsg=warning  WriteAfterWriteMsg=warning  WriteAfterReadMsg=warning  InitialValue=[0 0 0 0 0 0 0 0]  ShowAdditionalParam=off  OutDataTypeStr=uint16
  Data Store Memory4 : DataStoreMemory  DataStoreName=pts2_fifo_0_vect  ReadBeforeWriteMsg=warning  WriteAfterWriteMsg=warning  WriteAfterReadMsg=warning  InitialValue=[0 0 0 0 0 0 0 0]  ShowAdditionalParam=off  OutDataTypeStr=uint16
  Data Store Read : DataStoreRead  DataStoreName=pts2_fifo_0_vect  DataStoreElements=pts2_fifo_0_vect(2)#pts2_fifo_0_vect(1)
  Data Store Read1 : DataStoreRead  DataStoreName=pts2_fifo_1_vect  DataStoreElements=pts2_fifo_1_vect(1)
  Data Store Read2 : DataStoreRead  DataStoreName=pts2_fifo_0_vect  DataStoreElements=pts2_fifo_0_vect(1)
  Data Store Write3 : DataStoreWrite  DataStoreName=pts2_fifo_0_vect
  Data Store Write5 : DataStoreWrite  DataStoreName=pts2_fifo_1_vect
  Divide : Product  Inputs=*/  OutDataTypeStr=single
  Divide1 : Product  Inputs=*//
  Freq_MC : Constant  Value=80000000  OutDataTypeStr=single
  Prescaler : Constant  Value=32  OutDataTypeStr=single
  Subsystem : Subsystem
  Subsystem_capture : Subsystem
  Terminator1 : Terminator
  Terminator2 : Terminator
  eTimer_ISR : mbd_mpc574x_ec_toolbox/Motor Control Blocks/eTIMER Blocks/eTimer_ISR_Handler  etimerModule=1  etimerInterrupt=Channel Interrupt  etimerChannel=3  etimerIsrPriority=14
      settings: SourceProductName=NXP Model-Based Design Toolbox for MPC57xx MCUs
  DC : Outport
  freq : Outport  Port=2
  wires:
  Subsystem/1(Out1) -> DC/1
  Divide/1 -> Subsystem/1(In1)
  Data Store Read/1 -> Add/1
  Divide1/1 -> freq/1
  Data Store Read2/1 -> Add1/2
  Add1/1 -> Divide/1
  Freq_MC/1 -> Divide1/1
  Data Store Read/2 -> Add/2
  Data Store Read1/1 -> Add1/1
  Add/1 -> Divide1/3, Divide/2
  Prescaler/1 -> Divide1/2
  eTimer_ISR/1 -> Subsystem_capture/Trigger
  Subsystem_capture/2(Out2) -> Data Store Write3/1
  Subsystem_capture/4(Out4) -> Data Store Write5/1
  Subsystem_capture/3(Out3) -> Terminator2/1
  Subsystem_capture/1(Out1) -> Terminator1/1
  eTimer_ISR/2 -> Subsystem_capture/1(In1)

== system ZT_VehCtrl_18B/SigIn/PWM/PWM_PTS3 ==
  Add : Sum  Inputs=+-  AccumDataTypeStr=single
  Add1 : Sum  Inputs=+-  AccumDataTypeStr=single
  Data Store Memory : DataStoreMemory  DataStoreName=pts3_pwm_cnt  ReadBeforeWriteMsg=warning  WriteAfterWriteMsg=warning  WriteAfterReadMsg=warning  ShowAdditionalParam=off  OutDataTypeStr=uint8
  Data Store Memory2 : DataStoreMemory  DataStoreName=pts3_fifo_1_vect  ReadBeforeWriteMsg=warning  WriteAfterWriteMsg=warning  WriteAfterReadMsg=warning  InitialValue=[0 0 0 0 0 0 0 0]  ShowAdditionalParam=off  OutDataTypeStr=uint16
  Data Store Memory4 : DataStoreMemory  DataStoreName=pts3_fifo_0_vect  ReadBeforeWriteMsg=warning  WriteAfterWriteMsg=warning  WriteAfterReadMsg=warning  InitialValue=[0 0 0 0 0 0 0 0]  ShowAdditionalParam=off  OutDataTypeStr=uint16
  Data Store Read : DataStoreRead  DataStoreName=pts3_fifo_0_vect  DataStoreElements=pts3_fifo_0_vect(2)#pts3_fifo_0_vect(1)
  Data Store Read1 : DataStoreRead  DataStoreName=pts3_fifo_1_vect  DataStoreElements=pts3_fifo_1_vect(1)
  Data Store Read2 : DataStoreRead  DataStoreName=pts3_fifo_0_vect  DataStoreElements=pts3_fifo_0_vect(1)
  Data Store Write3 : DataStoreWrite  DataStoreName=pts3_fifo_0_vect
  Data Store Write5 : DataStoreWrite  DataStoreName=pts3_fifo_1_vect
  Divide : Product  Inputs=*/  OutDataTypeStr=single
  Divide1 : Product  Inputs=*//
  Freq_MC : Constant  Value=80000000  OutDataTypeStr=single
  Prescaler : Constant  Value=32  OutDataTypeStr=single
  Subsystem : Subsystem
  Subsystem_capture : Subsystem
  Terminator1 : Terminator
  Terminator2 : Terminator
  eTimer_ISR : mbd_mpc574x_ec_toolbox/Motor Control Blocks/eTIMER Blocks/eTimer_ISR_Handler  etimerModule=1  etimerInterrupt=Channel Interrupt  etimerChannel=1  etimerIsrPriority=14
      settings: SourceProductName=NXP Model-Based Design Toolbox for MPC57xx MCUs
  DC : Outport
  freq : Outport  Port=2
  wires:
  eTimer_ISR/2 -> Subsystem_capture/1(In1)
  Subsystem_capture/1(Out1) -> Terminator1/1
  Subsystem_capture/3(Out3) -> Terminator2/1
  Subsystem_capture/4(Out4) -> Data Store Write5/1
  Subsystem_capture/2(Out2) -> Data Store Write3/1
  eTimer_ISR/1 -> Subsystem_capture/Trigger
  Prescaler/1 -> Divide1/2
  Add/1 -> Divide/2, Divide1/3
  Data Store Read1/1 -> Add1/1
  Data Store Read/2 -> Add/2
  Freq_MC/1 -> Divide1/1
  Add1/1 -> Divide/1
  Data Store Read2/1 -> Add1/2
  Divide1/1 -> freq/1
  Data Store Read/1 -> Add/1
  Divide/1 -> Subsystem/1(In1)
  Subsystem/1(Out1) -> DC/1

== system ZT_VehCtrl_18B/SigIn/PWM/PWM_PTS4 ==
  Add : Sum  Inputs=+-  AccumDataTypeStr=single
  Add1 : Sum  Inputs=+-  AccumDataTypeStr=single
  Data Store Memory : DataStoreMemory  DataStoreName=pts4_pwm_cnt  ReadBeforeWriteMsg=warning  WriteAfterWriteMsg=warning  WriteAfterReadMsg=warning  ShowAdditionalParam=off  OutDataTypeStr=uint8
  Data Store Memory2 : DataStoreMemory  DataStoreName=pts4_fifo_1_vect  ReadBeforeWriteMsg=warning  WriteAfterWriteMsg=warning  WriteAfterReadMsg=warning  InitialValue=[0 0 0 0 0 0 0 0]  ShowAdditionalParam=off  OutDataTypeStr=uint16
  Data Store Memory4 : DataStoreMemory  DataStoreName=pts4_fifo_0_vect  ReadBeforeWriteMsg=warning  WriteAfterWriteMsg=warning  WriteAfterReadMsg=warning  InitialValue=[0 0 0 0 0 0 0 0]  ShowAdditionalParam=off  OutDataTypeStr=uint16
  Data Store Read : DataStoreRead  DataStoreName=pts4_fifo_0_vect  DataStoreElements=pts4_fifo_0_vect(2)#pts4_fifo_0_vect(1)
  Data Store Read1 : DataStoreRead  DataStoreName=pts4_fifo_1_vect  DataStoreElements=pts4_fifo_1_vect(1)
  Data Store Read2 : DataStoreRead  DataStoreName=pts4_fifo_0_vect  DataStoreElements=pts4_fifo_0_vect(1)
  Data Store Write3 : DataStoreWrite  DataStoreName=pts4_fifo_0_vect
  Data Store Write5 : DataStoreWrite  DataStoreName=pts4_fifo_1_vect
  Divide : Product  Inputs=*/  OutDataTypeStr=single
  Divide1 : Product  Inputs=*//
  Freq_MC : Constant  Value=80000000  OutDataTypeStr=single
  Prescaler : Constant  Value=32  OutDataTypeStr=single
  Subsystem : Subsystem
  Subsystem_capture : Subsystem
  Terminator1 : Terminator
  Terminator2 : Terminator
  eTimer_ISR : mbd_mpc574x_ec_toolbox/Motor Control Blocks/eTIMER Blocks/eTimer_ISR_Handler  etimerModule=0  etimerInterrupt=Channel Interrupt  etimerChannel=2  etimerIsrPriority=14
      settings: SourceProductName=NXP Model-Based Design Toolbox for MPC57xx MCUs
  DC : Outport
  freq : Outport  Port=2
  wires:
  Subsystem/1(Out1) -> DC/1
  Divide/1 -> Subsystem/1(In1)
  Data Store Read/1 -> Add/1
  Divide1/1 -> freq/1
  Data Store Read2/1 -> Add1/2
  Add1/1 -> Divide/1
  Freq_MC/1 -> Divide1/1
  Data Store Read/2 -> Add/2
  Data Store Read1/1 -> Add1/1
  Add/1 -> Divide1/3, Divide/2
  Prescaler/1 -> Divide1/2
  eTimer_ISR/1 -> Subsystem_capture/Trigger
  Subsystem_capture/2(Out2) -> Data Store Write3/1
  Subsystem_capture/4(Out4) -> Data Store Write5/1
  Subsystem_capture/3(Out3) -> Terminator2/1
  Subsystem_capture/1(Out1) -> Terminator1/1
  eTimer_ISR/2 -> Subsystem_capture/1(In1)

== system ZT_VehCtrl_18B/SigIn/PWM/Subsystem ==
  Data Store Memory1 : DataStoreMemory  DataStoreName=fifo_1_value  ReadBeforeWriteMsg=warning  WriteAfterWriteMsg=warning  WriteAfterReadMsg=warning  VectorParams1D=off  ShowAdditionalParam=off  OutDataTypeStr=uint16
  Data Store Memory3 : DataStoreMemory  DataStoreName=fifo_0_value  ReadBeforeWriteMsg=warning  WriteAfterWriteMsg=warning  WriteAfterReadMsg=warning  VectorParams1D=off  ShowAdditionalParam=off  OutDataTypeStr=uint16
  Data Store Memory5 : DataStoreMemory  DataStoreName=frequency  ReadBeforeWriteMsg=warning  WriteAfterWriteMsg=warning  WriteAfterReadMsg=warning  VectorParams1D=off  ShowAdditionalParam=off  OutDataTypeStr=single
  Data Store Memory6 : DataStoreMemory  DataStoreName=duty_cycle  ReadBeforeWriteMsg=warning  WriteAfterWriteMsg=warning  WriteAfterReadMsg=warning  VectorParams1D=off  ShowAdditionalParam=off  OutDataTypeStr=single
  Data Store Write10 : DataStoreWrite  DataStoreName=fifo_0_vect
  Data Store Write11 : DataStoreWrite  DataStoreName=fifo_1_value
  Data Store Write12 : DataStoreWrite  DataStoreName=fifo_1_vect
  Data Store Write13 : DataStoreWrite  DataStoreName=duty_cycle
  Data Store Write8 : DataStoreWrite  DataStoreName=frequency
  Data Store Write9 : DataStoreWrite  DataStoreName=fifo_0_value
  Frequency_DutyCycle_Computation : Subsystem
  eTimer Configuration and Signal Measurements : Subsystem
  wires:
  eTimer Configuration and Signal Measurements/4(Out4) -> Data Store Write12/1
  eTimer Configuration and Signal Measurements/2(Out2) -> Data Store Write10/1
  eTimer Configuration and Signal Measurements/3(Out3) -> Data Store Write11/1
  eTimer Configuration and Signal Measurements/1(Out1) -> Data Store Write9/1
  Frequency_DutyCycle_Computation/2(Out2) -> Data Store Write8/1
  Frequency_DutyCycle_Computation/1(Out1) -> Data Store Write13/1

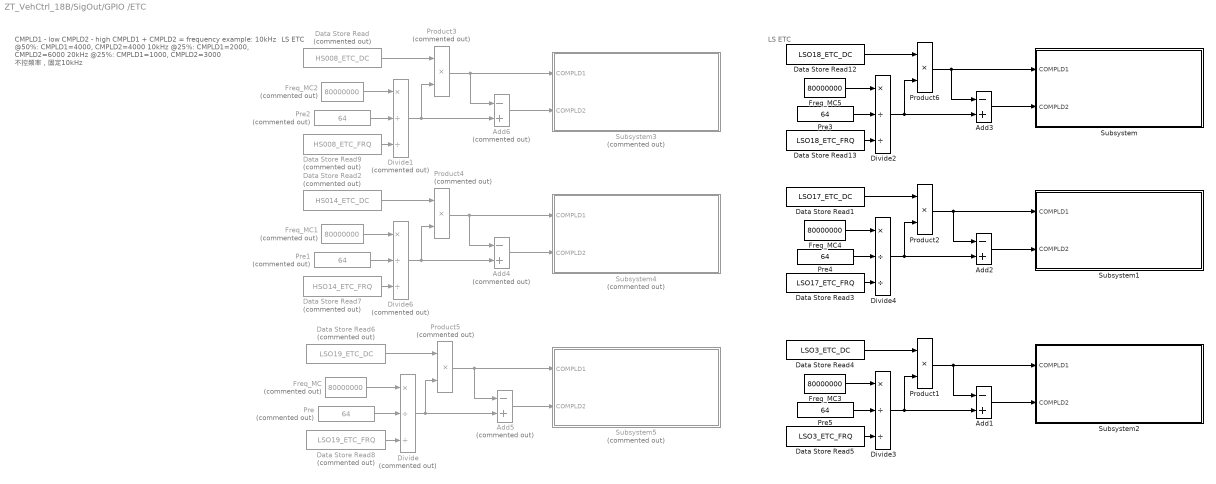
== system ZT_VehCtrl_18B/SigOut/GPIO /ETC ==
  note: CMPLD1 - low
      | CMPLD2 - high
      | CMPLD1 + CMPLD2 = frequency
      | example:
      | 10kHz @50%: CMPLD1=4000, CMPLD2=4000
      | 10kHz @25%: CMPLD1=2000, CMPLD2=6000
      | 20kHz @25%: CMPLD1=1000, CMPLD2=3000
      |
      | 不控频率，固定10kHz
  note: LS ETC
  note: LS ETC
  Add1 : Sum  Inputs=-+
  Add2 : Sum  Inputs=-+
  Add3 : Sum  Inputs=-+
  Add4 : Sum  Commented=on  Inputs=-+
  Add5 : Sum  Commented=on  Inputs=-+
  Add6 : Sum  Commented=on  Inputs=-+
  Data Store Read : DataStoreRead  Commented=on  DataStoreName=HS008_ETC_DC
  Data Store Read1 : DataStoreRead  DataStoreName=LSO17_ETC_DC
  Data Store Read12 : DataStoreRead  DataStoreName=LSO18_ETC_DC
  Data Store Read13 : DataStoreRead  DataStoreName=LSO18_ETC_FRQ
  Data Store Read2 : DataStoreRead  Commented=on  DataStoreName=HS014_ETC_DC
  Data Store Read3 : DataStoreRead  DataStoreName=LSO17_ETC_FRQ
  Data Store Read4 : DataStoreRead  DataStoreName=LSO3_ETC_DC
  Data Store Read5 : DataStoreRead  DataStoreName=LSO3_ETC_FRQ
  Data Store Read6 : DataStoreRead  Commented=on  DataStoreName=LSO19_ETC_DC
  Data Store Read7 : DataStoreRead  Commented=on  DataStoreName=HSO14_ETC_FRQ
  Data Store Read8 : DataStoreRead  Commented=on  DataStoreName=LSO19_ETC_FRQ
  Data Store Read9 : DataStoreRead  Commented=on  DataStoreName=HS008_ETC_FRQ
  Divide : Product  Commented=on  Inputs=*//
  Divide1 : Product  Commented=on  Inputs=*//
  Divide2 : Product  Inputs=*//
  Divide3 : Product  Inputs=*//
  Divide4 : Product  Inputs=*//
  Divide6 : Product  Commented=on  Inputs=*//
  Freq_MC : Constant  Commented=on  Value=80000000  OutDataTypeStr=single
  Freq_MC1 : Constant  Commented=on  Value=80000000  OutDataTypeStr=single
  Freq_MC2 : Constant  Commented=on  Value=80000000  OutDataTypeStr=single
  Freq_MC3 : Constant  Value=80000000  OutDataTypeStr=single
  Freq_MC4 : Constant  Value=80000000  OutDataTypeStr=single
  Freq_MC5 : Constant  Value=80000000  OutDataTypeStr=single
  Pre : Constant  Commented=on  Value=64
  Pre1 : Constant  Commented=on  Value=64
  Pre2 : Constant  Commented=on  Value=64
  Pre3 : Constant  Value=64
  Pre4 : Constant  Value=64
  Pre5 : Constant  Value=64
  Product1 : Product
  Product2 : Product
  Product3 : Product  Commented=on
  Product4 : Product  Commented=on
  Product5 : Product  Commented=on
  Product6 : Product
  Subsystem : Subsystem
  Subsystem1 : Subsystem
  Subsystem2 : Subsystem
  Subsystem3 : Subsystem  Commented=on
  Subsystem4 : Subsystem  Commented=on
  Subsystem5 : Subsystem  Commented=on
  wires:
  Data Store Read6/1 -> Product5/1
  Product5/1 -> Add5/1, Subsystem5/1(COMPLD1)
  Add5/1 -> Subsystem5/2(COMPLD2)
  Add4/1 -> Subsystem4/2(COMPLD2)
  Data Store Read8/1 -> Divide/3
  Data Store Read2/1 -> Product4/1
  Freq_MC/1 -> Divide/1
  Divide/1 -> Product5/2, Add5/2
  Divide6/1 -> Product4/2, Add4/2
  Freq_MC1/1 -> Divide6/1
  Data Store Read7/1 -> Divide6/3
  Product4/1 -> Add4/1, Subsystem4/1(COMPLD1)
  Divide1/1 -> Product3/2, Add6/2
  Freq_MC2/1 -> Divide1/1
  Data Store Read9/1 -> Divide1/3
  Product3/1 -> Add6/1, Subsystem3/1(COMPLD1)
  Data Store Read/1 -> Product3/1
  Add6/1 -> Subsystem3/2(COMPLD2)
  Divide3/1 -> Product1/2, Add1/2
  Freq_MC3/1 -> Divide3/1
  Data Store Read5/1 -> Divide3/3
  Product1/1 -> Add1/1, Subsystem2/1(COMPLD1)
  Divide4/1 -> Product2/2, Add2/2
  Freq_MC4/1 -> Divide4/1
  Data Store Read3/1 -> Divide4/3
  Product2/1 -> Add2/1, Subsystem1/1(COMPLD1)
  Divide2/1 -> Product6/2, Add3/2
  Freq_MC5/1 -> Divide2/1
  Data Store Read13/1 -> Divide2/3
  Product6/1 -> Add3/1, Subsystem/1(COMPLD1)
  Data Store Read1/1 -> Product2/1
  Data Store Read4/1 -> Product1/1
  Data Store Read12/1 -> Product6/1
  Add1/1 -> Subsystem2/2(COMPLD2)
  Add2/1 -> Subsystem1/2(COMPLD2)
  Add3/1 -> Subsystem/2(COMPLD2)
  Pre/1 -> Divide/2
  Pre1/1 -> Divide6/2
  Pre2/1 -> Divide1/2
  Pre3/1 -> Divide2/2
  Pre4/1 -> Divide4/2
  Pre5/1 -> Divide3/2
